simulink library "idealSensorProcessing_cl"  (R2022a)
settings: Solver=VariableStepAuto  StartTime=0.0  StopTime=10.0  RelTol=1e-3
undefined symbols (not defined in the file or in its folder): initializeBussesFromBlock
settings Model: Creator=mcobb  LastModifiedBy=adabney
settings SolverCC: AlgebraicLoopSolver=TrustRegion
settings DebuggingCC: UnconnectedInputMsg=warning  UnconnectedOutputMsg=warning  UnconnectedLineMsg=warning  SFMachineParentedDataDiag=warning  ArithmeticOperatorsInVariantConditions=warning
settings SFSimCC: CustomCodeUndefinedFunction=UseInterfaceOnly

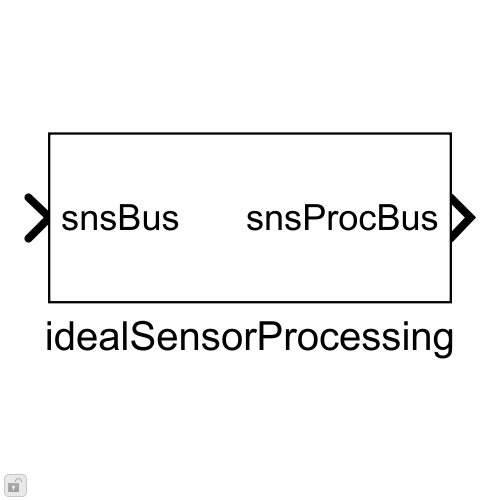
[thumbnail: Simulink's stored preview of the top-level diagram]
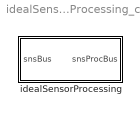
== system idealSensorProcessing_cl ==
  idealSensorProcessing : Subsystem  LoadFcn=initializeBussesFromBlock(gcb)  InitFcn=initializeBussesFromBlock(gcb)  StartFcn=initializeBussesFromBlock(gcb)

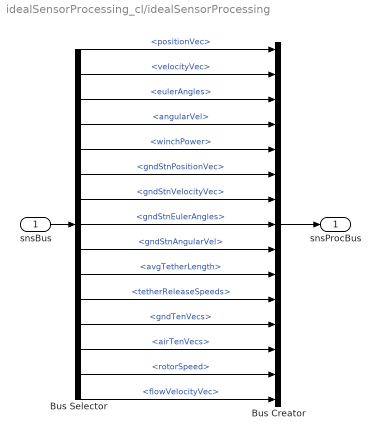
== system idealSensorProcessing_cl/idealSensorProcessing ==
  snsBus : Inport  OutDataTypeStr=Bus: sensorsBus
  Bus Creator : BusCreator  Inputs=15  OutDataTypeStr=Bus: sensorsProcessingBus  NonVirtualBus=on
  Bus Selector : BusSelector  OutputSignals=positionVec,velocityVec,eulerAngles,angularVel,winchPower,gndStnPositionVec,gndStnVelocityVec,gndStnEulerAngles,gndStnAngularVel,avgTetherLength,tetherReleaseSpeeds,gndTenVecs,airTenVecs,rotorSpeed,flowVelocityVec
  snsProcBus : Outport  OutDataTypeStr=Bus: sensorsProcessingBus  VectorParamsAs1DForOutWhenUnconnected=off
  wires:
  snsBus/1 -> Bus Selector/1
  Bus Creator/1 -> snsProcBus/1
  Bus Selector/1 -> Bus Creator/1  "<positionVec>"
  Bus Selector/2 -> Bus Creator/2  "<velocityVec>"
  Bus Selector/3 -> Bus Creator/3  "<eulerAngles>"
  Bus Selector/4 -> Bus Creator/4  "<angularVel>"
  Bus Selector/5 -> Bus Creator/5  "<winchPower>"
  Bus Selector/6 -> Bus Creator/6  "<gndStnPositionVec>"
  Bus Selector/7 -> Bus Creator/7  "<gndStnVelocityVec>"
  Bus Selector/8 -> Bus Creator/8  "<gndStnEulerAngles>"
  Bus Selector/9 -> Bus Creator/9  "<gndStnAngularVel>"
  Bus Selector/10 -> Bus Creator/10  "<avgTetherLength>"
  Bus Selector/11 -> Bus Creator/11  "<tetherReleaseSpeeds>"
  Bus Selector/12 -> Bus Creator/12  "<gndTenVecs>"
  Bus Selector/15 -> Bus Creator/15  "<flowVelocityVec>"
  Bus Selector/13 -> Bus Creator/13  "<airTenVecs>"
  Bus Selector/14 -> Bus Creator/14  "<rotorSpeed>"
